simulink model "chap7_6sim"  (Simulink 7.7)
settings: Solver=ode45  StartTime=0.0  StopTime=10  RelTol=1e-5
settings Model: Creator=hp  LastModifiedBy=ljk  ExtModeTrigMode=oneshot  ExtModeArmWhenConnect=off
settings DataIOCC: LimitDataPoints=off  SignalLoggingName=sigsOut
settings OptimizationCC: BooleanDataType=off  InitFltsAndDblsToZero=on
settings DebuggingCC: SaveWithParameterizedLinksMsg=none  SignalResolutionControl=TryResolveAllWithWarning  SolverPrmCheckMsg=none  MultiTaskDSMMsg=warning  MultiTaskCondExecSysMsg=none  StrictBusMsg=Warning
settings HardwareCC: TargetUnknown=on
settings RTWCC: IncludeERTFirstTime=on
settings GRTTargetCC: TargetFcnLib=ansi_tfl_tmw.mat

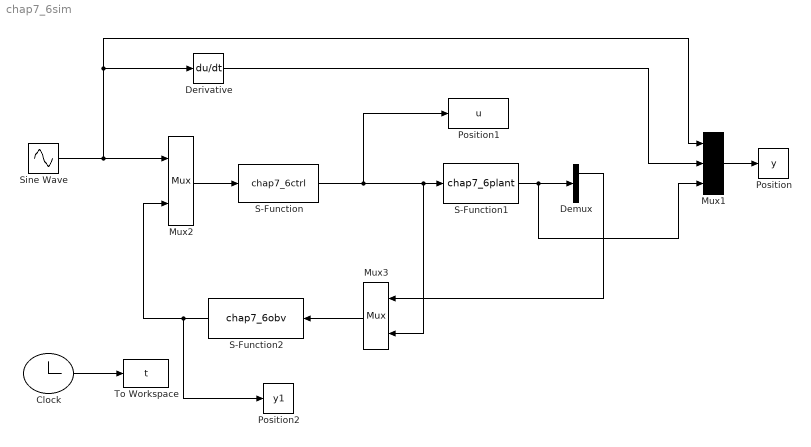
== system chap7_6sim ==
  Clock : Clock
      settings: Decimation=10
  Demux : Demux  Outputs=2
  Derivative : Derivative
  Mux1 : Mux  Inputs=3
  Mux2 : Mux  Inputs=2
  Mux3 : Mux  Inputs=2
  Position : ToWorkspace  VariableName=y  SampleTime=-1  SaveFormat=Array
  Position1 : ToWorkspace  VariableName=u  SampleTime=-1  SaveFormat=Array
  Position2 : ToWorkspace  VariableName=y1  SampleTime=-1  SaveFormat=Array
  S-Function : S-Function  FunctionName=chap7_6ctrl  EnableBusSupport=off
  S-Function1 : S-Function  FunctionName=chap7_6plant  EnableBusSupport=off
  S-Function2 : S-Function  FunctionName=chap7_6obv  EnableBusSupport=off
  Sine Wave : Sin  SampleTime=0
  To Workspace : ToWorkspace  VariableName=t  SampleTime=-1  SaveFormat=Array
  wires:
  Mux1/1 -> Position/1
  Clock/1 -> To Workspace/1
  Sine Wave/1 -> Mux2/1, Mux1/1, Derivative/1
  Mux2/1 -> S-Function/1
  S-Function/1 -> Position1/1, S-Function1/1, Mux3/2
  Derivative/1 -> Mux1/2
  Mux3/1 -> S-Function2/1
  Demux/1 -> Mux3/1
  S-Function1/1 -> Demux/1, Mux1/3
  S-Function2/1 -> Mux2/2, Position2/1
